simulink model "decouverte_filtrage"  (R2020b)
settings: Solver=FixedStepAuto  StartTime=0.0  StopTime=inf  RelTol=1e-3
PreLoadFcn:
  | f0=10
  | fs=1e3*f0
InitFcn:
  | f0=10
  | fs=1e3*f0
libraries: dspfdesign x2, dsparch4 x1, dspsrcs4 x1
settings Model: Creator=cmuller  LastModifiedBy=cmuller
settings SolverCC: AutoInsertRateTranBlk=on
settings DataIOCC: LimitDataPoints=on  SaveOutput=off  SignalLogging=off  SaveTime=off
settings OptimizationCC: LifeSpan=inf  SimCompilerOptimization=on
settings DebuggingCC: AlgebraicLoopMsg=error  SingleTaskRateTransMsg=error  AllowSymbolicDim=off  SFUnexpectedBacktrackingDiag=warning  SFNoUnconditionalDefaultTransitionDiag=warning  SFExecutionAtInitializationDiag=none  ArithmeticOperatorsInVariantConditions=warning
settings SFSimCC: SimUseLocalCustomCode=off  CustomCodeUndefinedFunction=UseInterfaceOnly
settings RTWCC: RTWUseLocalCustomCode=off
settings CodeAppCC: StateflowObjectComments=on
settings GRTTargetCC: TargetLangStandard=C89/C90 (ANSI)
settings ConfigComp: CovMetricSettings=dw  CovSaveCumulativeToWorkspaceVar=on  CovSaveSingleToWorkspaceVar=on  CovExternalEMLEnable=off  CovSFcnEnable=off

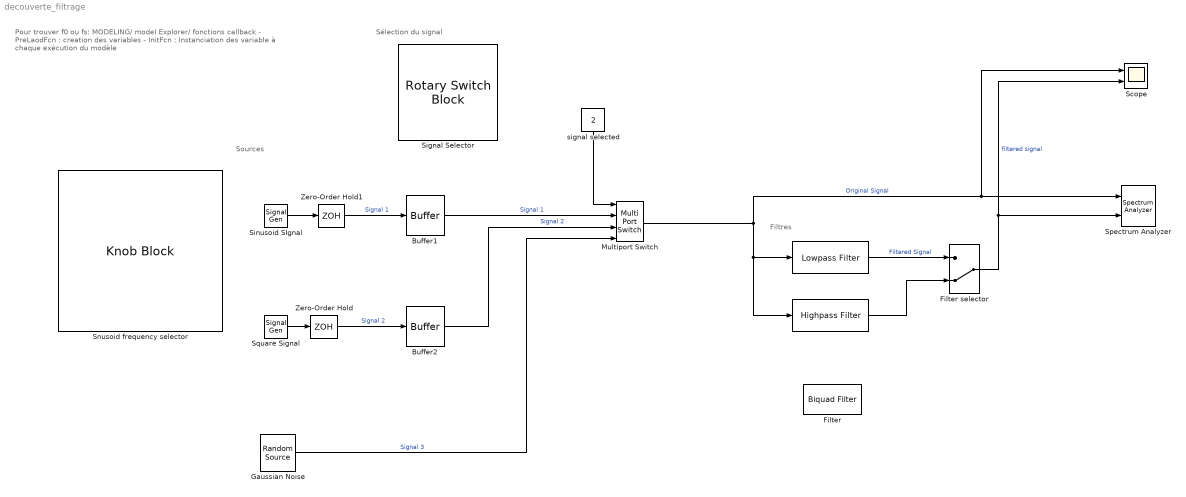
== system decouverte_filtrage ==
  note: Pour trouver f0 ou fs: MODELING/ model Explorer/ fonctions callback
      | - PreLaodFcn : creation des variables
      | - InitFcn : Instanciation des variable à chaque exécution du modèle
  note: Sélection du signal
  note: Sources
  note: Filtres
  " " : dspfdesign/Lowpass Filter  FilterType=IIR  DesignForMinimumOrder=on  FilterOrder=50  PassbandFrequency=4*f0  StopbandFrequency=5*f0  PassbandRipple=0.1  StopbandAttenuation=80  InheritSampleRate=off  SampleRate=fs  SimulateUsing=Code generation  roundingMode=Floor  coeffsDataTypeStr=fixdt(1,16)  mask(dsp.LowpassFilter){}
      mask Display:
      | % This is a new mask on top of the base mask.
      | % Use "View base mask" link below to see the base mask.
      | disp('Filtre 1')
  "  " : dspfdesign/Highpass Filter  FilterType=IIR  DesignForMinimumOrder=on  FilterOrder=50  StopbandFrequency=14*f0  PassbandFrequency=15*f0  StopbandAttenuation=80  PassbandRipple=0.1  InheritSampleRate=off  SampleRate=fs  SimulateUsing=Interpreted execution  roundingMode=Floor  coeffsDataTypeStr=fixdt(1,16)  mask(dsp.HighpassFilter){}
      mask Display:
      | % This is a new mask on top of the base mask.
      | % Use "View base mask" link below to see the base mask.
      | disp('Filtre 2')
  Buffer1 : Buffer  N=256  OutputFrames=off
  Buffer2 : Buffer  N=256  OutputFrames=off
  Filter : dsparch4/Biquad Filter  Tag=BlockMethodSubSystem  FilterSource=Dialog parameters  CoeffSource=Specify via dialog  FilterObject=BQF  IIRFiltStruct=Direct form II  BiQuadCoeffs=[1 0 -1 1 -1.99625341371283183 0.99912597641012324;1 0 -1 1 -1.99825402568306143 0.999438576140136203;1 0 -1 1 -1.99452405830929247 0.997387465358762215;1 0 -1 1 -1.99713079323974774 0.998317433242269181;1 0 -1 1 -1.99282589162178736 0.995673601544033393;1 0 -1 1 -1.99600836203715293 0.99719985479984119;1 0 -1 1 -1.99117277360844724 0.993998407689118402;1 0 -1 1 -1.99488834291324757 0.99608747166694811;1 0 -1 1 -1.98957803706871461 0.992375438869851134;1 0 -1 1 -1.99377248452741362 0.994982063708992115;1 0 -1 1 -1.98805434986085561 0.99081764223715818;1 0 -1 1 -1.99266273706356434 0.993885622645527489;1 0 -1 1 -1.98661358141934219 0.989337220542723661;1 0 -1 1 -1.99156131660078906 0.9928004151769102;1 0 -1 1 -1.98526667399032219 0.98794549983816693;1 0 -1 1 -1.99047076981142901 0.991729046017718163;1 0 -1 1 -1.98402351948006395 0.986652802171079091;1 0 -1 1 -1.98939403810509319 0.990674519923039343;1 0 -1 1 -1.98289284335248484 0.985468324715967126;1 0 -1 1 -1.98833451973924613 0.989640301113237086;1 0 -1 1 -1.98188209767657963 0.984400027370886277;1 0 -1 1 -1.98729612770434683 0.988630367868210791;1 0 -1 1 -1.98099736608560217 0.983454531511422592;1 0 -1 1 -1.98628334049196864 0.987649259388624912;1 0 -1 1 -1.9802432842880151 0.982637033572835716;1 0 -1 1 -1.98530124194566149 0.986702111061433573;1 0 -1 1 -1.97962298041625973 0.981951237752865747;1 0 -1 1 -1.9843555457275901 0.985794673703235369;1 0 -1 1 -1.97913803978795322 0.981399312463050899;1 0 -1 1 -1.98345259963232956 0.984933312114969262;1 0 -1 1 -1.97878849890818587 0.980981875504966516;1 0 -1 1 -1.98259936472054044 0.984124978060374245;1 0 -1 1 -1.97857287291578787 0.980698012367583583;1 0 -1 1 -1.98180336487352404 0.983377153512414615;1 0 -1 1 -1.97848821997568081 0.980545331494893313;1 0 -1 1 -1.98107260307976762 0.982697760713911128;1 0 -1 1 -1.97853024363610652 0.980520057812148904;1 0 -1 1 -1.98041544326335694 0.982095038301218692;1 0 -1 1 -1.97869343238511597 0.980617164159849231;1 0 -1 1 -1.97984045826874988 0.981577384470653791;1 0 -1 1 -1.9789712323071591 0.98083053692359834;1 0 -1 1 -1.97935624797507659 0.981153171556494397]  ScaleValues=[0.00959810193718166164;0.00959810193718166164;0.00959124212357875816;0.00959124212357875816;0.00958445441097437872;0.00958445441097437872;0.00957777622204819198;0.00957777622204819198;0.00957124414231682978;0.00957124414231682978;0.00956489373364006329;0.00956489373364006329;0.0095587593578222059;0.0095587593578222059;0.00955287401075316858;0.00955287401075316858;0.00954726916740343198;0.00954726916740343198;0.00954197463787007788;0.00954197463787007788;0.00953701843456801826;0.00953701843456801826;0.0095324266505724415;0.0095324266505724415;0.0095282233490456246;0.0095282233490456246;0.00952443046362363467;0.00952443046362363467;0.00952106770959576;0.00952106770959576;0.00951815250568109616;0.00951815250568109616;0.00951569990619185319;0.00951569990619185319;0.00951372254337046371;0.00951372254337046371;0.00951223057969631004;0.00951223057969631004;0.00951123166997639921;0.00951123166997639921;0.00951073093306131247;0.00951073093306131247;1]  IC=0  ICnum=0  ICden=0  a0Flag=Warning  optimizeScaleValues=on  ScaleValueMode=Specify via input port (g)  InputProcessing=Columns as channels (frame based)  roundingMode=Floor  overflowMode=off  scaleValueFracLength=14  denProdOutputFracLength=30  denAccumFracLength=30  secondMemoryFracLength=15  mask(Biquad Filter){}
      mask Display:
      | % This is a new mask on top of the base mask.
      | % Use "View base mask" link below to see the base mask.
      | disp('Unknown filter')
  Filter selector : ManualSwitch  CurrentSetting=0
  Gaussian Noise : dspsrcs4/Random Source  SrcType=Gaussian  NormMethod=Ziggurat  CltLength=12  MinVal=0  MaxVal=1  MeanVal=0  VarVal=.05  RepMode=Specify seed  rawSeed=1234567  IsInherit=off  SampMode=Discrete  SampTime=1/fs  SampFrame=256  DataType=Double  OutComplex=Real  OutputFrames=off
  Multiport Switch : MultiPortSwitch  DiagnosticForDefault=None
  Scope : Scope  NumInputPorts=2
  Signal Selector : RotarySwitchBlock  LabelPosition=Hide
      settings: Values={{'sig1', 'sig2', 'sig3'}, [1 2 3]}
  Sinusoid SIgnal : SignalGenerator  Frequency=31.4653205871582
  Snusoid frequency selector : KnobBlock  Description=Signal selector  ScaleMax=250
  Spectrum Analyzer : SpectrumAnalyzer  NumInputPorts=2
  Square Signal : SignalGenerator  WaveForm=square  Frequency=f0
  Zero-Order Hold : ZeroOrderHold  SampleTime=1/fs
  Zero-Order Hold1 : ZeroOrderHold  SampleTime=1/fs
  signal selected : Constant  Value=2  SampleTime=-1
  wires:
  Multiport Switch/1 -> Scope/1, Spectrum Analyzer/1, "  "/1, " "/1  "Original Signal"
  " "/1 -> Filter selector/1  "Filtered Signal"
  Filter selector/1 -> Scope/2, Spectrum Analyzer/2  "filtered signal"
  Square Signal/1 -> Zero-Order Hold/1
  signal selected/1 -> Multiport Switch/1
  Zero-Order Hold/1 -> Buffer2/1  "Signal 2"
  Sinusoid SIgnal/1 -> Zero-Order Hold1/1
  Zero-Order Hold1/1 -> Buffer1/1  "Signal 1"
  Gaussian Noise/1 -> Multiport Switch/4  "Signal 3"
  Buffer1/1 -> Multiport Switch/2  "Signal 1"
  Buffer2/1 -> Multiport Switch/3  "Signal 2"
  "  "/1 -> Filter selector/2
